simulink model "mpc_model_dual_module_resistiveLoad"  (R2019a)
settings: Solver=FixedStepAuto  StartTime=0.0  StopTime=Tfinal  RelTol=1e-3
values from neighbouring files (symbols this model uses):
  A = [-0.0285 -0.0014; -0.0371 -0.1476]    [model.m]
  DCLINK_Cap = 1000e-12    (= 1e-09)    [mpc_model_parameters.m]    (also in mpc_model_parameters_dual_module.m = 0.001)
  FluxPM = MeanInducedVoltagePeak/(2*pi*100)    [mpc_model_parameters.m]    (also in mpc_model_parameters_dual_module.m)
  Inertia = 1e-2    (= 0.01)    [mpc_model_parameters.m]    (also in mpc_model_parameters_dual_module.m)
  iqrated = Trated/(1.5*PolePairs*FluxPM)    [mpc_model_parameters.m]    (also in mpc_model_parameters_dual_module.m)
  Ki = 8    [mpc_model_parameters_dual_module.m]
  Kp = 0.8    [mpc_model_parameters_dual_module.m]
  Ls = 3.5e-3    (= 0.0035)    [MPC_id_iq.m]    (also in mpc_model_parameters.m = 0.00351; mpc_model_parameters_dual_module.m = 0.00343)
  M1_FaultTime = 0.25    [mpc_model_parameters_dual_module.m]
  MeanLd = (1/12)*(Module1Phase_A_Ld+Module1Phase_B_Ld+Module1Phase_C_Ld+     Module2Phase_A_Ld+Module2Phase_B_Ld+Module2Phase_C_Ld+     Module3Phase_A_Ld+Module3Phase_B_Ld+Module3Phase_C_Ld+     Module4Phase_A_Ld+Module4Phase_B_Ld+Module4Phase_C_Ld)    [mpc_model_parameters.m]    (also in mpc_model_parameters_dual_module.m)
  MeanLq = (1/12)*(Module1Phase_A_Lq+Module1Phase_B_Lq+Module1Phase_C_Lq+     Module2Phase_A_Lq+Module2Phase_B_Lq+Module2Phase_C_Lq+     Module3Phase_A_Lq+Module3Phase_B_Lq+Module3Phase_C_Lq+     Module4Phase_A_Lq+Module4Phase_B_Lq+Module4Phase_C_Lq)    [mpc_model_parameters.m]    (also in mpc_model_parameters_dual_module.m)
  PI_Frequency = 5000    [mpc_model_parameters_dual_module.m]
  PI_Sat = iqrated*2    [mpc_model_parameters_dual_module.m]
  PI_Ts = 1/PI_Frequency    (= 0.0002)    [mpc_model_parameters_dual_module.m]
  PolePairs = 10    [mpc_model_parameters.m]    (also in mpc_model_parameters_dual_module.m)
  RefModeSelection = 1    [mpc_model_parameters_dual_module.m]
  Rin = 1e-3    (= 0.001)    [mpc_model_parameters.m]    (also in mpc_model_parameters_dual_module.m)
  Rs = 0.531    [Loss_Distribution.m]    (also in MPC_id_iq.m; mpc_model_parameters.m = 0.321; mpc_model_parameters_dual_module.m = 0.539)
  Sampling_time = 1e-6    (= 1e-06)    [mpc_model_parameters.m]    (also in mpc_model_parameters_dual_module.m)
  SpeedRef1 = 50    [mpc_model_parameters.m]    (also in mpc_model_parameters_dual_module.m = 35)
  SpeedRef2 = 100    [mpc_model_parameters.m]    (also in mpc_model_parameters_dual_module.m = 35)
  SpeedRefUpdateTime = 0.25    [mpc_model_parameters.m]    (also in mpc_model_parameters_dual_module.m = 1.75)
  Tload1 = 5    [mpc_model_parameters.m]    (also in mpc_model_parameters_dual_module.m = 30)
  Tload2 = 10    [mpc_model_parameters.m]    (also in mpc_model_parameters_dual_module.m = 63.6619772368)
  TloadUpdateTime = 0.5    [mpc_model_parameters.m]    (also in mpc_model_parameters_dual_module.m)
  Vdc = 50    [mpc_model_parameters.m]    (also in mpc_model_parameters_dual_module.m = 40)
  Vin = Vdc + Rin*(Pout/Vdc)    (= 50.04)    [mpc_model_parameters.m]    (also in mpc_model_parameters_dual_module.m = 40.05)
  ViscousFriction = 1e-3    (= 0.001)    [mpc_model_parameters.m]    (also in mpc_model_parameters_dual_module.m)
undefined symbols (not defined in the file or in its folder): DiscIntNeverNeededParam, FaultTolerantControlTime, LoadResistance1, LoadResistance2, VoltageConstant_omega
libraries: powerlib x37, dspsigops x28, dspswit3 x19, powerlib_meascontrol x11, fl_lib x5, simulink x4, nesl_utility x3, sdl_lib x1
(part 3 of 3)

== matlab function mpc_model_dual_module_resistiveLoad/M1 Prediction ==
  data: p1_out output; p2_out output; p3_out output; p4_out output; p5_out output; DutyA output; DutyB output; DutyC output; iqref input; idref input; IdMeasured input; IqMeasured input; Ls input; Rs input; PolePairs input; wref input; ShaftAngularSpeed input; FluxPM input; Vdc input; ElectricalAngle input; InterruptPulse input; DutyA_prev input; DutyB_prev input; DutyC_prev input; SimulationClock input; FaultOccuranceTime input; FswSelected_prev input; FswSelected output; IqRipplePrediction output; IqRipplePrediction_prev input; Speed_Error_prev input; Speed_Error output; Vds_Optimum output; Vqs_Optimum output; Vds_Optimum_prev input; Vqs_Optimum_prev input; filter_out_prev input; filter_out output
function [p1_out, p2_out, p3_out, p4_out, p5_out,DutyA, DutyB, DutyC, FswSelected, IqRipplePrediction,Speed_Error,Vds_Optimum,Vqs_Optimum,filter_out] = fcn(iqref,idref,IdMeasured, IqMeasured,  Ls, Rs,PolePairs,wref, ShaftAngularSpeed, FluxPM,Vdc,ElectricalAngle,InterruptPulse,DutyA_prev, DutyB_prev, DutyC_prev, SimulationClock,FaultOccuranceTime,FswSelected_prev, IqRipplePrediction_prev,Speed_Error_prev,Vds_Optimum_prev,Vqs_Optimum_prev,filter_out_prev)
Ld = Ls;
Lq = Ls;
Iq_Rated = 11.7362; %this is the rated value of the IqMeasured
% cost = zeros(1,8);
% VdPrediction_1 = zeros(1,8);
% VqPrediction_1 = zeros(1,8);
% FswOptions = [5000; 10000; 15000; 20000; 25000; 30000; 35000; 40000];
FswMax = 10000;
FswOptions = 1000:1000:FswMax;
cost = zeros(1,numel(FswOptions));
% VdPrediction_1 = zeros(1,numel(FswOptions));
% VqPrediction_1 = zeros(1,numel(FswOptions));
Vd_est_1 = zeros(1,numel(FswOptions));
Vq_est_1 = zeros(1,numel(FswOptions));
% Vd_est_2 = zeros(1,numel(FswOptions));
% Vq_est_2 = zeros(1,numel(FswOptions));
VdPrediction_2 = zeros(1,numel(FswOptions));
VqPrediction_2 = zeros(1,numel(FswOptions));
IqRipplePredictionArray_1 = zeros(1,numel(FswOptions));
IqRipplePredictionArray_2 = zeros(1,numel(FswOptions));
VoltageDuring_T1_1 = zeros(1,numel(FswOptions));
VoltageDuring_T2_1 = zeros(1,numel(FswOptions));
VoltageDuring_T0_1 = zeros(1,numel(FswOptions));
VoltageDuring_T1_2 = zeros(1,numel(FswOptions));
VoltageDuring_T2_2 = zeros(1,numel(FswOptions));
VoltageDuring_T0_2 = zeros(1,numel(FswOptions));
MagnitudePrediction_1 = zeros(1,numel(FswOptions));
MagnitudePrediction_2 = zeros(1,numel(FswOptions));

SvpwmT1Prediction_1 =  zeros(1,numel(FswOptions));
SvpwmT2Prediction_1 =  zeros(1,numel(FswOptions));
SvpwmT0Prediction_1 =  zeros(1,numel(FswOptions));

SvpwmT1Prediction_2 =  zeros(1,numel(FswOptions));
SvpwmT2Prediction_2 =  zeros(1,numel(FswOptions));
SvpwmT0Prediction_2 =  zeros(1,numel(FswOptions));

ValfaPrediction_1 = zeros(1,numel(FswOptions)); 
VbetaPrediction_1 = zeros(1,numel(FswOptions)); 
ValfaPrediction_2 = zeros(1,numel(FswOptions)); 
VbetaPrediction_2 = zeros(1,numel(FswOptions)); 
maPrediction_1 = zeros(1,numel(FswOptions)); 
maPrediction_2 = zeros(1,numel(FswOptions));

IqDelta_Prediction_During_T1_1 =  zeros(1,numel(FswOptions));
IqDelta_Prediction_During_T2_1 =  zeros(1,numel(FswOptions));
IqDelta_Prediction_During_T0_1 =  zeros(1,numel(FswOptions));
IqDelta_Prediction_During_T1_2 =  zeros(1,numel(FswOptions));
IqDelta_Prediction_During_T2_2 =  zeros(1,numel(FswOptions));
IqDelta_Prediction_During_T0_2 =  zeros(1,numel(FswOptions));
VoltageVectorAnglePredictionMod_1 = zeros(1,numel(FswOptions));
VoltageVectorAnglePrediction_1 = zeros(1,numel(FswOptions));
VoltageVectorAnglePredictionMod_2 = zeros(1,numel(FswOptions));
VoltageVectorAnglePrediction_2 = zeros(1,numel(FswOptions));

IdPrediction_1_array = zeros(1,numel(FswOptions));
IqPrediction_1_array = zeros(1,numel(FswOptions));
IdPrediction_2_array = zeros(1,numel(FswOptions));
IqPrediction_2_array = zeros(1,numel(FswOptions));

p1 = zeros(1,numel(FswOptions));
p2 = zeros(1,numel(FswOptions));
p3 = zeros(1,numel(FswOptions));
p4 = zeros(1,numel(FswOptions));
p5 = zeros(1,numel(FswOptions));

p1_out = 0;
p2_out = 0;
p3_out = 0;
p4_out = 0;
p5_out = 0;


Vd_Vq_Kp = 10;
Vd_Vq_Ki = 1;

MinimumCostValue = 1e20;
MinimumCostIndex = -1;

% IqRippleCoeff = 100000;
% IqRefCoeff = 10000;
% IdRefCoeff = 15;
% FswCoeff = 1250;

IqRippleCoeff = 100000;
IqRefCoeff = 1000000;
IdRefCoeff = 1000000;
FswCoeff = 1250;
FswInertiaCoeff = 750;


Iq_1_Method1 = 0;
Id_1_Method1 = 0;
Iq_2_Method1 = 0;
Id_2_Method1 = 0;
Kp = 0.35;
Ki = 50;
Ts_PI = 1/40000;
OptimizeForFsws = 0;
if(FswSelected_prev<=0)
    FswSelected_prev = 1000;
end
% % % % % % % % if((FswSelected_prev==1000)||(FswSelected_prev==2000))
% % % % % % % %     OptimizeForFsws = 1:1:5;
% % % % % % % % else if((FswSelected_prev==10000)||(FswSelected_prev==9000))
% % % % % % % %      OptimizeForFsws = 5:1:10;
% % % % % % % %     else
% % % % % % % %         OptimizeForFsws = (FswSelected_prev/1000-2):1:(FswSelected_prev/1000+2);
% % % % % % % %     end
% % % % % % % % end
if(FswSelected_prev==1000)
    OptimizeForFsws = 1:1:2;
else if(FswSelected_prev==10000)
     OptimizeForFsws = 9:1:10;
    else
        OptimizeForFsws = (FswSelected_prev/1000-1):1:(FswSelected_prev/1000+1);
    end
end

Speed_Error =  wref-ShaftAngularSpeed;
Speed_Error_RPM = Speed_Error/(2*pi)*60;

% deriv_speed = (ShaftAngularSpeed - ShaftAngularSpeed_prev)* FswSelected_prev;

if((abs(Speed_Error_RPM)>5)||(abs(filter_out_prev/100)>5))
    %         OptimizeForFsws(3) = 10;
    %         OptimizeForFsws(2) = 9;
    % IqRippleCoeff = 100000;
    IqRefCoeff = 1000000*100;
    IdRefCoeff = 1000000*100;
    % FswCoeff = 2500/5;
else
    IqRippleCoeff = 100000;
    IqRefCoeff = 1000000;
    IdRefCoeff = 1000000;
    FswCoeff = 4500;
end

% y = y_prev + Kp*(u-u_prev)+Ts/2*Ki*(u+u_prev);
if(InterruptPulse==1)
    Speed_Error =  wref-ShaftAngularSpeed;
    filter_out = filter_out_prev + Speed_Error_RPM;
    filter_out = filter_out - filter_out/100;    
%     iqref = iqref_prev + Kp*(Speed_Error-Speed_Error_prev)+Ts_PI/2*Ki*((Speed_Error+Speed_Error_prev));
% 
%     if(abs(iqref)>(2*Iq_Rated))
%         if(iqref>0)
%             iqref = (2*Iq_Rated);
%         else
%             iqref = -(2*Iq_Rated);
%         end
%     end
%     for i = 1:numel(FswOptions)
    for i = OptimizeForFsws(1):OptimizeForFsws(end)

        IdPrediction_1 = IdMeasured + (0.5/FswSelected_prev + 0.5/FswOptions(i))*(Vds_Optimum_prev/Ld-Rs/Ld*IdMeasured+Lq/Ld*PolePairs*ShaftAngularSpeed*IqMeasured);
        IqPrediction_1 = IqMeasured + (0.5/FswSelected_prev + 0.5/FswOptions(i))*(Vqs_Optimum_prev/Lq-Rs/Lq*IqMeasured-Ld/Lq*PolePairs*ShaftAngularSpeed*IdMeasured-FluxPM*PolePairs*ShaftAngularSpeed/Lq);
        
                
        IdPrediction_1_array(i) = IdPrediction_1;
        IqPrediction_1_array(i) = IqPrediction_1;
        
        Vd_Vq_Kp = Ls/(2)*FswOptions(i);
        Vd_Vq_Ki = Rs/Ls;
        
        Vd_est_1(i) = Vd_Vq_Kp * (idref-IdPrediction_1) * ( 1 + Vd_Vq_Ki / FswOptions(i) ) + IdMeasured - PolePairs*ShaftAngularSpeed*Ls*IqPrediction_1;
        Vq_est_1(i) = Vd_Vq_Kp * (iqref-IqPrediction_1) * ( 1 + Vd_Vq_Ki / FswOptions(i) ) + IqMeasured + PolePairs*ShaftAngularSpeed*(Ls*IdPrediction_1 + FluxPM);

        
     
        
        %% second prediction
        
        
        MagnitudePrediction_2(i) = sqrt(Vd_est_1(i)^2+Vq_est_1(i)^2);
        
        ValfaPrediction_2(i) = sin(ElectricalAngle)*Vd_est_1(i)+cos(ElectricalAngle)*Vq_est_1(i);
        VbetaPrediction_2(i) =-cos(ElectricalAngle)*Vd_est_1(i)+sin(ElectricalAngle)*Vq_est_1(i);      
        
        VoltageVectorAnglePrediction_2(i) = atan2(VbetaPrediction_2(i),ValfaPrediction_2(i))+4*pi;%(PolePairs*ShaftAngularSpeed/FswOptions(i));
        VoltageVectorAnglePredictionMod_2(i) = mod(VoltageVectorAnglePrediction_2(i),pi/3);   
        
        maPrediction_2(i) = MagnitudePrediction_2(i)/(Vdc/sqrt(3)); 
        
        if(SimulationClock>FaultOccuranceTime)
%             IqRefCoeff = 100;
            SvpwmT1Prediction_2(i) = (1/FswOptions(i))*maPrediction_2(i)*sin(mod(VoltageVectorAnglePrediction_2(i),pi));
            SvpwmT2Prediction_2(i) = 0;
            SvpwmT0Prediction_2(i) = (1/FswOptions(i))-SvpwmT1Prediction_2(i)-SvpwmT2Prediction_2(i);       
%             IdRefCoeff = 100;
        else
            SvpwmT1Prediction_2(i) = (1/FswOptions(i))*maPrediction_2(i)*sin(pi/3-VoltageVectorAnglePredictionMod_2(i));
            SvpwmT2Prediction_2(i) = (1/FswOptions(i))*maPrediction_2(i)*sin(VoltageVectorAnglePredictionMod_2(i));
            SvpwmT0Prediction_2(i) = (1/FswOptions(i))-SvpwmT1Prediction_2(i)-SvpwmT2Prediction_2(i);    
        end  
        
        VoltageDuring_T1_2(i) = 2/3*Vdc-MagnitudePrediction_2(i);
        VoltageDuring_T2_2(i) = 2/3*Vdc-MagnitudePrediction_2(i);
        VoltageDuring_T0_2(i) = -MagnitudePrediction_2(i);
        
        IqDelta_Prediction_During_T1_2(i) = -VoltageDuring_T1_2(i)*SvpwmT1Prediction_2(i)/Ls;
        IqDelta_Prediction_During_T2_2(i) = -VoltageDuring_T2_2(i)*SvpwmT2Prediction_2(i)/Ls;
        IqDelta_Prediction_During_T0_2(i) = VoltageDuring_T0_2(i)*SvpwmT0Prediction_2(i)/Ls;        
        
        IqRipplePredictionArray_2(i) = IqDelta_Prediction_During_T1_2(i)+IqDelta_Prediction_During_T2_2(i)+IqDelta_Prediction_During_T0_2(i);
        
        IdPrediction_2 = IdPrediction_1 + (1/FswOptions(i))*(Vd_est_1(i)/Ld-Rs/Ld*IdPrediction_1+Lq/Ld*PolePairs*ShaftAngularSpeed*IqPrediction_1);
        IqPrediction_2 = IqPrediction_1 + (1/FswOptions(i))*(Vq_est_1(i)/Lq-Rs/Lq*IqPrediction_1-Ld/Lq*PolePairs*ShaftAngularSpeed*IdPrediction_1-FluxPM*PolePairs*ShaftAngularSpeed/Lq);                
        
        IdPrediction_2_array(i) = IdPrediction_2;
        IqPrediction_2_array(i) = IqPrediction_2;
        

        ProtectionConstant = 0;
%         cost(i) = FswInertiaCoeff*abs(FswSelected_prev-FswOptions(i))/FswMax+(IqRipplePredictionArray_2(i)/Iq_Rated)^2*IqRippleCoeff+IqRefCoeff*((iqref-IqPrediction_2)/Iq_Rated)^2+((idref-IdPrediction_2)/Iq_Rated)^2*IdRefCoeff+ProtectionConstant+FswOptions(i)/FswMax*FswCoeff;%+IqRipplePrediction_prev^2*100000000;

p1(i) = FswInertiaCoeff*abs(FswSelected_prev-FswOptions(i))/FswMax;
p2(i) = (IqRipplePredictionArray_2(i)/Iq_Rated)^2*IqRippleCoeff;
p3(i) = IqRefCoeff*((iqref-IqPrediction_2)/Iq_Rated)^2;
p4(i) = ((idref-IdPrediction_2)/Iq_Rated)^2*IdRefCoeff;
p5(i) = FswOptions(i)/FswMax*FswCoeff;
        cost(i) = p1(i) + p2(i) + p3(i) + p4(i) + p5(i);
        
        
        if(cost(i)<MinimumCostValue)
            MinimumCostValue = cost(i);
            MinimumCostIndex = i;
        end
        
    end
    
%     [CostMinVal, MinimumCostIndex] = min(cost);

p1_out = p1(MinimumCostIndex);
p2_out = p2(MinimumCostIndex);
p3_out = p3(MinimumCostIndex);
p4_out = p4(MinimumCostIndex);
p5_out = p5(MinimumCostIndex);

    DutyA = 0;
    DutyB = 0;
    DutyC = 0;
    VdsOptimum_1 = VdPrediction_2(MinimumCostIndex);
    VqsOptimum_1 = VqPrediction_2(MinimumCostIndex);
    FswSelected = FswOptions(MinimumCostIndex);
    
    Iq_1_Method1 = IqPrediction_1_array(MinimumCostIndex);
    Id_1_Method1 = IdPrediction_1_array(MinimumCostIndex);

    Iq_2_Method1 = IqPrediction_2_array(MinimumCostIndex);
    Id_2_Method1 = IdPrediction_2_array(MinimumCostIndex);
    
    VoltageVectorAngleOptimum = VoltageVectorAnglePrediction_2(MinimumCostIndex);
    TswSelected = 1/FswSelected;
    
    Vds_Optimum = Vd_est_1(MinimumCostIndex);
    Vqs_Optimum = Vq_est_1(MinimumCostIndex);

    
    Svpwm_T1 = SvpwmT1Prediction_2(MinimumCostIndex);
    Svpwm_T2 = SvpwmT2Prediction_2(MinimumCostIndex);
    Svpwm_T0 = SvpwmT0Prediction_2(MinimumCostIndex);
    
    IqRipplePrediction = IqRipplePredictionArray_2(MinimumCostIndex);
    
    if(SimulationClock>FaultOccuranceTime)
        if (mod(VoltageVectorAngleOptimum, 2*pi)<=pi)  
            DutyB = (Svpwm_T1+Svpwm_T0/2)/TswSelected;
            DutyC = (Svpwm_T0/2)/TswSelected;
        else
            DutyC = (Svpwm_T1+Svpwm_T0/2)/TswSelected;
            DutyB = (Svpwm_T0/2)/TswSelected;
        end
        DutyA = 0;
        return;
    end        
    
    if (mod(VoltageVectorAngleOptimum, 2*pi)<=pi/3)&&(mod(VoltageVectorAngleOptimum, 2*pi)>=0)  % sector 1
        DutyA = (Svpwm_T1+Svpwm_T2+Svpwm_T0/2)/TswSelected;
        DutyB = (Svpwm_T2+Svpwm_T0/2)/TswSelected;
        DutyC = (Svpwm_T0/2)/TswSelected;
%         sectornumber = 1;
        return;
    end
    if (mod(VoltageVectorAngleOptimum, 2*pi)<=2*pi/3)&&(mod(VoltageVectorAngleOptimum, 2*pi)>=pi/3)  % sector 2
        DutyA = (Svpwm_T1+Svpwm_T0/2)/TswSelected;
        DutyB = (Svpwm_T1+Svpwm_T2+Svpwm_T0/2)/TswSelected;
        DutyC = (Svpwm_T0/2)/TswSelected;
%         sectornumber = 2;
        return;
    end
    if (mod(VoltageVectorAngleOptimum, 2*pi)<=pi)&&(mod(VoltageVectorAngleOptimum, 2*pi)>=2*pi/3)  % sector 3
        if(mod(VoltageVectorAngleOptimum, pi)==0)
            DutyA = (Svpwm_T0/2)/TswSelected;
            DutyB = (Svpwm_T1+Svpwm_T0/2)/TswSelected;
            DutyC = (Svpwm_T1+Svpwm_T2+Svpwm_T0/2)/TswSelected;
        else
            DutyA = (Svpwm_T0/2)/TswSelected;
            DutyB = (Svpwm_T1+Svpwm_T2+Svpwm_T0/2)/TswSelected;
            DutyC = (Svpwm_T2+Svpwm_T0/2)/TswSelected;
        end
%         sectornumber = 3;
        return;
    end
    if (mod(VoltageVectorAngleOptimum, 2*pi)<=4*pi/3)&&(mod(VoltageVectorAngleOptimum, 2*pi)>=pi)  % sector 4
        DutyA = (Svpwm_T0/2)/TswSelected;
        DutyB = (Svpwm_T1+Svpwm_T0/2)/TswSelected;
        DutyC = (Svpwm_T1+Svpwm_T2+Svpwm_T0/2)/TswSelected;
%         sectornumber = 4;
        return;
    end
    if (mod(VoltageVectorAngleOptimum, 2*pi)<=5*pi/3)&&(mod(VoltageVectorAngleOptimum, 2*pi)>=4*pi/3)  % sector 5
        DutyA = (Svpwm_T2+Svpwm_T0/2)/TswSelected;
        DutyB = (Svpwm_T0/2)/TswSelected;
        DutyC = (Svpwm_T1+Svpwm_T2+Svpwm_T0/2)/TswSelected;
%         sectornumber = 5;
        return;
    end
    if (mod(VoltageVectorAngleOptimum, 2*pi)<=2*pi)&&(mod(VoltageVectorAngleOptimum, 2*pi)>=5*pi/3)  % sector 6
        DutyA = (Svpwm_T1+Svpwm_T2+Svpwm_T0/2)/TswSelected;
        DutyB = (Svpwm_T0/2)/TswSelected;
        DutyC = (Svpwm_T1+Svpwm_T0/2)/TswSelected;
%         sectornumber = 6;
        return;
    end
    
else %switching pulse
%     iqref = iqref_prev;
    Speed_Error = Speed_Error_prev;
    FswSelected = FswSelected_prev;
    DutyA = DutyA_prev;
    DutyB = DutyB_prev;
    DutyC = DutyC_prev;
    IqRipplePrediction = IqRipplePrediction_prev;
    Vds_Optimum = Vds_Optimum_prev;
    Vqs_Optimum = Vqs_Optimum_prev;
    filter_out = filter_out_prev;    
end

== matlab function mpc_model_dual_module_resistiveLoad/MATLAB Function1 ==
  data: pulse input; inputwave input; outputwave output
function outputwave  = fcn(pulse, inputwave)

persistent state

if isempty(state)
state = 0;
end

if(pulse==1)
    state = state +1;
end

if(mod(state,2)==1)
    outputwave = inputwave;
    return;
end
if(mod(state,2)==0)
    outputwave = 1-inputwave;
    return;
end

outputwave = 5;

== matlab function mpc_model_dual_module_resistiveLoad/MATLAB Function2 ==
  data: pulse input; inputwave input; outputwave output
function outputwave  = fcn(pulse, inputwave)

persistent state

if isempty(state)
state = 0;
end

if(pulse==1)
    state = state +1;
end

if(mod(state,2)==1)
    outputwave = inputwave;
    return;
end
if(mod(state,2)==0)
    outputwave = 1-inputwave;
    return;
end

outputwave = 5;

== matlab function mpc_model_dual_module_resistiveLoad/module 1 abc to dq1 ==
  data: ids output; iqs output; ias input; ibs input; ics input; ref_frame_position input; i0 output
function [ids,iqs,i0 ]  = fcn(ias,ibs,ics,ref_frame_position)





ids = 2/3*(ias*sin(ref_frame_position)+ibs*sin(ref_frame_position-2*pi/3)+ics*sin(ref_frame_position+2*pi/3));
iqs =  2/3*(ias*cos(ref_frame_position)+ibs*cos(ref_frame_position-2*pi/3)+ics*cos(ref_frame_position+2*pi/3));
i0 = 2/3*1/2*(ias+ibs+ics);
% iqs = (vqs-fluxlinkage_qs_derivative-ref_frame_velocity*fluxlinkage_ds)/rs;
% ids = (vds-fluxlinkage_ds_derivative+ref_frame_velocity*fluxlinkage_qs)/rs;

== matlab function mpc_model_dual_module_resistiveLoad/MATLAB Function4 ==
  data: M1_ia input; M1_loss output; M1_ib input; M1_ic input; M2_ia input; M2_ib input; M2_ic input; M2_loss output; Total_loss output; Rs input
function [M1_loss,M2_loss,Total_loss] = fcn(M1_ia, M1_ib, M1_ic, M2_ia, M2_ib, M2_ic, Rs)



M1_loss = Rs*(M1_ia^2+M1_ib^2+M1_ic^2);
M2_loss = Rs*(M2_ia^2+M2_ib^2+M2_ic^2);
Total_loss = M1_loss+M2_loss;

== matlab function mpc_model_dual_module_resistiveLoad/MATLAB Function5 ==
  data: M1_ids input; M1_magnetic_loss output; M1_iqs input; M2_ids input; M2_iqs input; FluxPM input; Ls input; ElectricalSpeed input; M2_magnetic_loss output; Total_loss output
function [M1_magnetic_loss,M2_magnetic_loss,Total_loss] = fcn(M1_ids,M1_iqs,M2_ids,M2_iqs,FluxPM,Ls,ElectricalSpeed)

cfe = 1.55;
lambda = 1.55;
M1_d_axis_flux = Ls*M1_ids+FluxPM;
M1_q_axis_flux = Ls*M1_iqs;
M2_d_axis_flux = Ls*M2_ids+FluxPM;
M2_q_axis_flux = Ls*M2_iqs;

M1_magnetic_loss = cfe*power(abs(ElectricalSpeed),lambda)*(M1_d_axis_flux^2+M1_q_axis_flux^2);
M2_magnetic_loss = cfe*power(abs(ElectricalSpeed),lambda)*(M2_d_axis_flux^2+M2_q_axis_flux^2);

% M1_loss = Rs*(M1_ia^2+M1_ib^2+M1_ic^2);
% M2_loss = Rs*(M2_ia^2+M2_ib^2+M2_ic^2);
Total_loss = M1_magnetic_loss+M2_magnetic_loss;

== matlab function mpc_model_dual_module_resistiveLoad/MATLAB Function6 ==
  data: pulse input; inputwave input; outputwave output
function outputwave  = fcn(pulse, inputwave)

persistent state

if isempty(state)
state = 0;
end

if(pulse==1)
    state = state +1;
end

if(mod(state,2)==1)
    outputwave = inputwave;
    return;
end
if(mod(state,2)==0)
    outputwave = 1-inputwave;
    return;
end

outputwave = 5;

== matlab function mpc_model_dual_module_resistiveLoad/MATLAB Function7 ==
  data: M1_Iq_opt_cost input; M1_iqref output; M1_Id_opt_cost input; M2_Iq_opt_cost input; M2_Id_opt_cost input; M1_Iq_opt_proportional input; M1_Id_opt_proportional input; M2_Iq_opt_proportional input; M2_Id_opt_proportional input; M1_Iq_opt_equal input; M1_Id_opt_equal input; M2_Iq_opt_equal input; M2_Id_opt_equal input; M1_idref output; M2_iqref output; M2_idref output; selection input
function [M1_iqref, M1_idref, M2_iqref, M2_idref] = fcn(M1_Iq_opt_cost,M1_Id_opt_cost,M2_Iq_opt_cost,M2_Id_opt_cost...
    ,M1_Iq_opt_proportional,M1_Id_opt_proportional,M2_Iq_opt_proportional,M2_Id_opt_proportional,...
    M1_Iq_opt_equal,M1_Id_opt_equal,M2_Iq_opt_equal,M2_Id_opt_equal,selection)


if(selection==1)
    M1_iqref = M1_Iq_opt_cost;
    M1_idref = M1_Id_opt_cost;
    M2_iqref = M2_Iq_opt_cost;
    M2_idref = M2_Id_opt_cost;
    return
end


if(selection==2)
    M1_iqref = M1_Iq_opt_proportional;
    M1_idref = M1_Id_opt_proportional;
    M2_iqref = M2_Iq_opt_proportional;
    M2_idref = M2_Id_opt_proportional;
    return
end



if(selection==3)
    M1_iqref = M1_Iq_opt_equal;
    M1_idref = M1_Id_opt_equal;
    M2_iqref = M2_Iq_opt_equal;
    M2_idref = M2_Id_opt_equal;
    return
end



    M1_iqref = M1_Iq_opt_equal;
    M1_idref = M1_Id_opt_equal;
    M2_iqref = M2_Iq_opt_equal;
    M2_idref = M2_Id_opt_equal;

== matlab function mpc_model_dual_module_resistiveLoad/MATLAB Function8 ==
  data: interrupt1 input; phase output; interrupt2 input; time1 input; time2 input; counter_prev input; counter output; phase_prev input
function [phase, counter ] = fcn(interrupt1, interrupt2,time1, time2,counter_prev,phase_prev)

counter_temp = counter_prev;
if(interrupt1 == 1)
    counter_temp = counter_temp +1;   
end

if(interrupt2 == 1)
    counter_temp = counter_temp +1;  
end

counter = counter_temp;

if(mod(counter,2)==1)
    phase = time1-time2;
else
    phase = phase_prev;
end

== matlab function mpc_model_dual_module_resistiveLoad/MATLAB Function10 ==
  data: pulse input; inputwave input; outputwave output
function outputwave  = fcn(pulse, inputwave)

persistent state

if isempty(state)
state = 0;
end

if(pulse==1)
    state = state +1;
end

if(mod(state,2)==1)
    outputwave = inputwave;
    return;
end
if(mod(state,2)==0)
    outputwave = 1-inputwave;
    return;
end

outputwave = 5;

== matlab function mpc_model_dual_module_resistiveLoad/MATLAB Function9 ==
  data: InterruptSignal input; Ref input; Measured input; Ki input; Output output; Kp input; Ts input; Sat input; Error output; ErrorPrev input; OutputPrev input
function [Output,Error] = fcn(InterruptSignal,Ref,Measured,Ki,Kp,Ts,Sat, ErrorPrev,OutputPrev)
Error=0;
Output = 0;

if(InterruptSignal ==1)
    Error = Ref-Measured;
    
    Output = OutputPrev + Kp*(Error-ErrorPrev)+Ts/2*Ki*((Error+ErrorPrev));
    %  iqref = iqref_prev + Kp*(Speed_Error-Speed_Error_prev)+Ts_PI/2*Ki*((Speed_Error+Speed_Error_prev));
    if(abs(Output)>(Sat))
        if(Output>0)
            Output = Sat;
        else
            Output = -(Sat);
        end
    end
else
    Output=OutputPrev;
    Error = ErrorPrev;
end

== matlab function mpc_model_dual_module_resistiveLoad/module 2 abc to dq1 ==
  data: ids output; iqs output; ias input; ibs input; ics input; ref_frame_position input; i0 output
function [ids,iqs,i0 ]  = fcn(ias,ibs,ics,ref_frame_position)





ids = 2/3*(ias*sin(ref_frame_position)+ibs*sin(ref_frame_position-2*pi/3)+ics*sin(ref_frame_position+2*pi/3));
iqs =  2/3*(ias*cos(ref_frame_position)+ibs*cos(ref_frame_position-2*pi/3)+ics*cos(ref_frame_position+2*pi/3));
i0 = 2/3*1/2*(ias+ibs+ics);
% iqs = (vqs-fluxlinkage_qs_derivative-ref_frame_velocity*fluxlinkage_ds)/rs;
% ids = (vds-fluxlinkage_ds_derivative+ref_frame_velocity*fluxlinkage_qs)/rs;

== matlab function mpc_model_dual_module_resistiveLoad/MATLAB Function12 ==
  data: M1_id input; M1_copper_loss output; M1_iq input; M2_id input; M2_iq input; M2_copper_loss output
function [M1_copper_loss, M2_copper_loss ] = fcn(M1_id, M1_iq, M2_id, M2_iq)

Rs = 0.539;

M1_copper_loss = 1.5*Rs*(M1_id^2+M1_iq^2);

M2_copper_loss = 1.5*Rs*(M2_id^2+M2_iq^2);

== matlab function mpc_model_dual_module_resistiveLoad/MATLAB Function13 ==
  data: Switch_Current input; fsw input; ConductionLoss output; SwitchingLoss output
function  [ConductionLoss, SwitchingLoss] = fcn(Switch_Current,fsw)

Rds_on = 2e-3;
GateCurrent = 1;

Qgs2 = 6.3e-9;
Qgd = 6.7e-9;

ConductionLoss = Rds_on*Switch_Current^2;
SwitchingLoss = 40*abs(Switch_Current)*fsw*(Qgs2+Qgd)/GateCurrent;
% y = u;

== matlab function mpc_model_dual_module_resistiveLoad/MATLAB Function14 ==
  data: Switch_Current input; fsw input; ConductionLoss output; SwitchingLoss output
function  [ConductionLoss, SwitchingLoss] = fcn(Switch_Current,fsw)

Rds_on = 2e-3;
GateCurrent = 1;

Qgs2 = 6.3e-9;
Qgd = 6.7e-9;

ConductionLoss = Rds_on*Switch_Current^2;
SwitchingLoss = 40*abs(Switch_Current)*fsw*(Qgs2+Qgd)/GateCurrent;
% y = u;

== matlab function mpc_model_dual_module_resistiveLoad/MATLAB Function15 ==
  data: moment1 input; phase output; moment2 input; fsw1 input
function phase = fcn(moment1,moment2,fsw1)

timedifference = moment2-moment1;

phase = timedifference*fsw1*360;

if(phase <0)
    phase = phase + 360;
end

% y = u;

== matlab function mpc_model_dual_module_resistiveLoad/MATLAB Function16 ==
  data: Switch_Current input; fsw input; ConductionLoss output; SwitchingLoss output
function  [ConductionLoss, SwitchingLoss] = fcn(Switch_Current,fsw)

Rds_on = 2e-3;
GateCurrent = 1;

Qgs2 = 6.3e-9;
Qgd = 6.7e-9;

ConductionLoss = Rds_on*Switch_Current^2;
SwitchingLoss = 40*abs(Switch_Current)*fsw*(Qgs2+Qgd)/GateCurrent;
% y = u;

== matlab function mpc_model_dual_module_resistiveLoad/MATLAB Function17 ==
  data: Switch_Current input; fsw input; ConductionLoss output; SwitchingLoss output
function  [ConductionLoss, SwitchingLoss] = fcn(Switch_Current,fsw)

Rds_on = 2e-3;
GateCurrent = 1;

Qgs2 = 6.3e-9;
Qgd = 6.7e-9;

ConductionLoss = Rds_on*Switch_Current^2;
SwitchingLoss = 40*abs(Switch_Current)*fsw*(Qgs2+Qgd)/GateCurrent;
% y = u;

== matlab function mpc_model_dual_module_resistiveLoad/MATLAB Function18 ==
  data: Switch_Current input; fsw input; ConductionLoss output; SwitchingLoss output
function  [ConductionLoss, SwitchingLoss] = fcn(Switch_Current,fsw)

Rds_on = 2e-3;
GateCurrent = 1;

Qgs2 = 6.3e-9;
Qgd = 6.7e-9;

ConductionLoss = Rds_on*Switch_Current^2;
SwitchingLoss = 40*abs(Switch_Current)*fsw*(Qgs2+Qgd)/GateCurrent;
% y = u;

== matlab function mpc_model_dual_module_resistiveLoad/MATLAB Function19 ==
  data: Switch_Current input; fsw input; ConductionLoss output; SwitchingLoss output
function  [ConductionLoss, SwitchingLoss] = fcn(Switch_Current,fsw)

Rds_on = 2e-3;
GateCurrent = 1;

Qgs2 = 6.3e-9;
Qgd = 6.7e-9;

ConductionLoss = Rds_on*Switch_Current^2;
SwitchingLoss = 40*abs(Switch_Current)*fsw*(Qgs2+Qgd)/GateCurrent;
% y = u;

== matlab function mpc_model_dual_module_resistiveLoad/MATLAB Function20 ==
  data: Switch_Current input; fsw input; ConductionLoss output; SwitchingLoss output
function  [ConductionLoss, SwitchingLoss] = fcn(Switch_Current,fsw)

Rds_on = 2e-3;
GateCurrent = 1;

Qgs2 = 6.3e-9;
Qgd = 6.7e-9;

ConductionLoss = Rds_on*Switch_Current^2;
SwitchingLoss = 40*abs(Switch_Current)*fsw*(Qgs2+Qgd)/GateCurrent;
% y = u;

== matlab function mpc_model_dual_module_resistiveLoad/MATLAB Function21 ==
  data: Switch_Current input; fsw input; ConductionLoss output; SwitchingLoss output
function  [ConductionLoss, SwitchingLoss] = fcn(Switch_Current,fsw)

Rds_on = 2e-3;
GateCurrent = 1;

Qgs2 = 6.3e-9;
Qgd = 6.7e-9;

ConductionLoss = Rds_on*Switch_Current^2;
SwitchingLoss = 40*abs(Switch_Current)*fsw*(Qgs2+Qgd)/GateCurrent;
% y = u;

== matlab function mpc_model_dual_module_resistiveLoad/MATLAB Function22 ==
  data: Switch_Current input; fsw input; ConductionLoss output; SwitchingLoss output
function  [ConductionLoss, SwitchingLoss] = fcn(Switch_Current,fsw)

Rds_on = 2e-3;
GateCurrent = 1;

Qgs2 = 6.3e-9;
Qgd = 6.7e-9;

ConductionLoss = Rds_on*Switch_Current^2;
SwitchingLoss = 40*abs(Switch_Current)*fsw*(Qgs2+Qgd)/GateCurrent;
% y = u;

== matlab function mpc_model_dual_module_resistiveLoad/MATLAB Function23 ==
  data: Switch_Current input; fsw input; ConductionLoss output; SwitchingLoss output
function  [ConductionLoss, SwitchingLoss] = fcn(Switch_Current,fsw)

Rds_on = 2e-3;
GateCurrent = 1;

Qgs2 = 6.3e-9;
Qgd = 6.7e-9;

ConductionLoss = Rds_on*Switch_Current^2;
SwitchingLoss = 40*abs(Switch_Current)*fsw*(Qgs2+Qgd)/GateCurrent;
% y = u;

== matlab function mpc_model_dual_module_resistiveLoad/MATLAB Function24 ==
  data: Switch_Current input; fsw input; ConductionLoss output; SwitchingLoss output
function  [ConductionLoss, SwitchingLoss] = fcn(Switch_Current,fsw)

Rds_on = 2e-3;
GateCurrent = 1;

Qgs2 = 6.3e-9;
Qgd = 6.7e-9;

ConductionLoss = Rds_on*Switch_Current^2;
SwitchingLoss = 40*abs(Switch_Current)*fsw*(Qgs2+Qgd)/GateCurrent;
% y = u;

== matlab function mpc_model_dual_module_resistiveLoad/MATLAB Function25 ==
  data: Switch_Current input; fsw input; ConductionLoss output; SwitchingLoss output
function  [ConductionLoss, SwitchingLoss] = fcn(Switch_Current,fsw)

Rds_on = 2e-3;
GateCurrent = 1;

Qgs2 = 6.3e-9;
Qgd = 6.7e-9;

ConductionLoss = Rds_on*Switch_Current^2;
SwitchingLoss = 40*abs(Switch_Current)*fsw*(Qgs2+Qgd)/GateCurrent;
% y = u;

== matlab function mpc_model_dual_module_resistiveLoad/Mechanical Subsystem/MATLAB Function ==
  data: u input; y output
function y = fcn(u)

if(abs(u)<=0.001)
    y = 0.1;
else 
    y = u;
end

% y = u;
